simulink library "MESSIN_Library"  (R2024a)
settings: Solver=VariableStepAuto  StartTime=0.0  StopTime=10.0  RelTol=1e-3
undefined symbols (not defined in the file or in its folder): actuatorCommand, commandedActuator, commandMode, externCommand, ready, remoteControlDevice, sensor, supervisor, timestampUTC, useXNAllocation
libraries: $bdroot x376, etargetslib x52, simulink x19
(part 2 of 5)

== system MESSIN_Library/State Message/Empty MESSIN State Bus/Empty INS Bus ==
  Bus Creator1 : BusCreator  Inputs=5
  Bus Creator2 : BusCreator  Inputs=17
  Constant1 : Constant  Value=0  OutDataTypeStr=uint8
  Constant{2..8,12..14,18..23} (16 alike) : Constant  Value=0.0  OutDataTypeStr=double
  Constant24 : Constant  Value=false  OutDataTypeStr=boolean
  Constant25 : Constant  Value=false  OutDataTypeStr=boolean
  Constant26 : Constant  Value=0  OutDataTypeStr=uint16
  Constant27 : Constant  Value=0  OutDataTypeStr=uint16
  Signal Specification1 : SignalSpecification  OutDataTypeStr=double  Unit=s  Dimensions=1
  Signal Specification{2..3,11..13} (5 alike) : SignalSpecification  OutDataTypeStr=double  Unit=rad  Dimensions=1
  Signal Specification17 : SignalSpecification  OutDataTypeStr=double  Unit=rad/s  Dimensions=1
  Signal Specification18 : SignalSpecification  OutDataTypeStr=double  Unit=rad/s  Dimensions=1
  Signal Specification19 : SignalSpecification  OutDataTypeStr=double  Unit=rad/s  Dimensions=1
  Signal Specification20 : SignalSpecification  OutDataTypeStr=double  Unit=m/s^2  Dimensions=1
  Signal Specification21 : SignalSpecification  OutDataTypeStr=double  Unit=m/s^2  Dimensions=1
  Signal Specification22 : SignalSpecification  OutDataTypeStr=double  Unit=m/s^2  Dimensions=1
  Signal Specification23 : SignalSpecification  OutDataTypeStr=uint8  Dimensions=1
  Signal Specification24 : SignalSpecification  OutDataTypeStr=boolean  Dimensions=1
  Signal Specification25 : SignalSpecification  OutDataTypeStr=boolean  Dimensions=1
  Signal Specification26 : SignalSpecification  OutDataTypeStr=uint16  Dimensions=1
  Signal Specification27 : SignalSpecification  OutDataTypeStr=uint16  Dimensions=1
  Signal Specification4 : SignalSpecification  OutDataTypeStr=double  Unit=m  Dimensions=1
  Signal Specification5 : SignalSpecification  OutDataTypeStr=double  Unit=m/s  Dimensions=1
  Signal Specification6 : SignalSpecification  OutDataTypeStr=double  Unit=m/s  Dimensions=1
  Signal Specification7 : SignalSpecification  OutDataTypeStr=double  Unit=m/s  Dimensions=1
  insLFK100 : Outport
  wires:
  Signal Specification1/1 -> Bus Creator2/1  "timestampUTC"
  Signal Specification6/1 -> Bus Creator2/6  "velocityEast"
  Constant4/1 -> Signal Specification3/1
  Constant19/1 -> Signal Specification18/1
  Signal Specification20/1 -> Bus Creator2/14  "bodyAccelerationX"
  Constant23/1 -> Signal Specification22/1
  Signal Specification13/1 -> Bus Creator2/10  "heading"
  Signal Specification2/1 -> Bus Creator2/2  "latitude"
  Constant14/1 -> Signal Specification13/1
  Bus Creator2/1 -> insLFK100/1
  Constant6/1 -> Signal Specification5/1
  Constant13/1 -> Signal Specification12/1
  Signal Specification11/1 -> Bus Creator2/8  "roll"
  Constant3/1 -> Signal Specification2/1
  Signal Specification12/1 -> Bus Creator2/9  "pitch"
  Signal Specification5/1 -> Bus Creator2/5  "velocityNorth"
  Signal Specification18/1 -> Bus Creator2/12  "bodyAngularRateY"
  Constant5/1 -> Signal Specification4/1
  Constant18/1 -> Signal Specification17/1
  Signal Specification3/1 -> Bus Creator2/3  "longitude"
  Signal Specification4/1 -> Bus Creator2/4  "heave"
  Constant20/1 -> Signal Specification19/1
  Constant12/1 -> Signal Specification11/1
  Constant2/1 -> Signal Specification1/1
  Signal Specification22/1 -> Bus Creator2/16  "bodyAccelerationZ"
  Signal Specification7/1 -> Bus Creator2/7  "velocityDown"
  Signal Specification19/1 -> Bus Creator2/13  "bodyAngularRateZ"
  Constant8/1 -> Signal Specification7/1
  Constant21/1 -> Signal Specification20/1
  Constant22/1 -> Signal Specification21/1
  Constant7/1 -> Signal Specification6/1
  Signal Specification17/1 -> Bus Creator2/11  "bodyAngularRateX"
  Signal Specification21/1 -> Bus Creator2/15  "bodyAccelerationY"
  Constant1/1 -> Signal Specification23/1
  Signal Specification27/1 -> Bus Creator1/5  "statusWord2"
  Signal Specification26/1 -> Bus Creator1/4  "statusWord1"
  Signal Specification25/1 -> Bus Creator1/3  "reducedAccuracy"
  Signal Specification24/1 -> Bus Creator1/2  "systemFailure"
  Signal Specification23/1 -> Bus Creator1/1  "mode"
  Constant24/1 -> Signal Specification24/1
  Constant25/1 -> Signal Specification25/1
  Constant26/1 -> Signal Specification26/1
  Constant27/1 -> Signal Specification27/1
  Bus Creator1/1 -> Bus Creator2/17  "details"

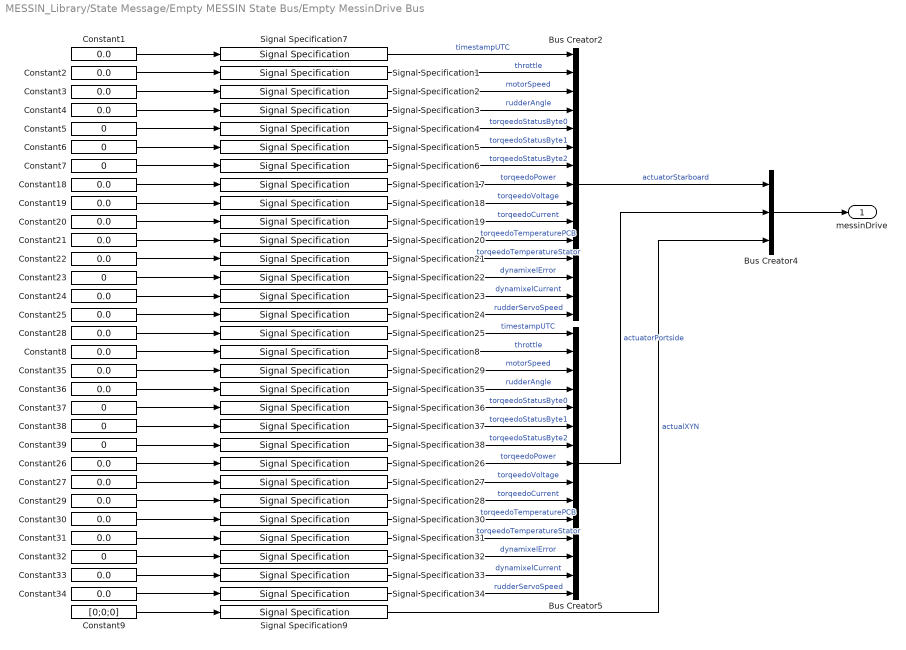
== system MESSIN_Library/State Message/Empty MESSIN State Bus/Empty MessinDrive Bus ==
  Bus Creator2 : BusCreator  Inputs=15
  Bus Creator4 : BusCreator  Inputs=3
  Bus Creator5 : BusCreator  Inputs=15
  Constant{1..4,8,18..22,24..31,33..36} (22 alike) : Constant  Value=0.0  OutDataTypeStr=double
  Constant{5..7,23,32,37..39} (8 alike) : Constant  Value=0  OutDataTypeStr=uint8
  Constant9 : Constant  Value=[0;0;0]  OutDataTypeStr=double
  Signal Specification1 : SignalSpecification  OutDataTypeStr=double  Unit=1  Dimensions=1
  Signal Specification17 : SignalSpecification  OutDataTypeStr=double  Unit=W  Dimensions=1
  Signal Specification18 : SignalSpecification  OutDataTypeStr=double  Unit=V  Dimensions=1
  Signal Specification{19,23,28,33} (4 alike) : SignalSpecification  OutDataTypeStr=double  Unit=A  Dimensions=1
  Signal Specification{2,24,29,34} (4 alike) : SignalSpecification  OutDataTypeStr=double  Unit=rad/s  Dimensions=1
  Signal Specification{20..21,30..31} (4 alike) : SignalSpecification  OutDataTypeStr=double  Unit=°C  Dimensions=1
  Signal Specification{4..6,22,32,36..38} (8 alike) : SignalSpecification  OutDataTypeStr=uint8  Unit=1  Dimensions=1
  Signal Specification25 : SignalSpecification  OutDataTypeStr=double  Unit=s  Dimensions=1
  Signal Specification26 : SignalSpecification  OutDataTypeStr=double  Unit=W  Dimensions=1
  Signal Specification27 : SignalSpecification  OutDataTypeStr=double  Unit=V  Dimensions=1
  Signal Specification3 : SignalSpecification  OutDataTypeStr=double  Unit=rad  Dimensions=1
  Signal Specification35 : SignalSpecification  OutDataTypeStr=double  Unit=rad  Dimensions=1
  Signal Specification7 : SignalSpecification  OutDataTypeStr=double  Unit=s  Dimensions=1
  Signal Specification8 : SignalSpecification  OutDataTypeStr=double  Unit=1  Dimensions=1
  Signal Specification9 : SignalSpecification  OutDataTypeStr=double  Dimensions=3
  messinDrive : Outport
  wires:
  Constant36/1 -> Signal Specification35/1
  Signal Specification1/1 -> Bus Creator2/2  "throttle"
  Signal Specification17/1 -> Bus Creator2/8  "torqeedoPower"
  Constant20/1 -> Signal Specification19/1
  Constant30/1 -> Signal Specification30/1
  Constant37/1 -> Signal Specification36/1
  Signal Specification25/1 -> Bus Creator5/1  "timestampUTC"
  Signal Specification4/1 -> Bus Creator2/5  "torqeedoStatusByte0"
  Signal Specification26/1 -> Bus Creator5/8  "torqeedoPower"
  Signal Specification2/1 -> Bus Creator2/3  "motorSpeed"
  Constant22/1 -> Signal Specification21/1
  Constant18/1 -> Signal Specification17/1
  Signal Specification5/1 -> Bus Creator2/6  "torqeedoStatusByte1"
  Constant25/1 -> Signal Specification24/1
  Signal Specification37/1 -> Bus Creator5/6  "torqeedoStatusByte1"
  Signal Specification21/1 -> Bus Creator2/12  "torqeedoTemperatureStator"
  Constant32/1 -> Signal Specification32/1
  Signal Specification36/1 -> Bus Creator5/5  "torqeedoStatusByte0"
  Constant2/1 -> Signal Specification1/1
  Constant5/1 -> Signal Specification4/1
  Signal Specification28/1 -> Bus Creator5/10  "torqeedoCurrent"
  Constant35/1 -> Signal Specification29/1
  Signal Specification19/1 -> Bus Creator2/10  "torqeedoCurrent"
  Signal Specification32/1 -> Bus Creator5/13  "dynamixelError"
  Constant7/1 -> Signal Specification6/1
  Constant21/1 -> Signal Specification20/1
  Signal Specification29/1 -> Bus Creator5/3  "motorSpeed"
  Signal Specification30/1 -> Bus Creator5/11  "torqeedoTemperaturePCB"
  Signal Specification38/1 -> Bus Creator5/7  "torqeedoStatusByte2"
  Bus Creator4/1 -> messinDrive/1
  Signal Specification22/1 -> Bus Creator2/13  "dynamixelError"
  Constant4/1 -> Signal Specification3/1
  Signal Specification35/1 -> Bus Creator5/4  "rudderAngle"
  Constant28/1 -> Signal Specification25/1
  Signal Specification20/1 -> Bus Creator2/11  "torqeedoTemperaturePCB"
  Signal Specification24/1 -> Bus Creator2/15  "rudderServoSpeed"
  Constant24/1 -> Signal Specification23/1
  Constant19/1 -> Signal Specification18/1
  Constant27/1 -> Signal Specification27/1
  Constant6/1 -> Signal Specification5/1
  Constant33/1 -> Signal Specification33/1
  Signal Specification18/1 -> Bus Creator2/9  "torqeedoVoltage"
  Constant29/1 -> Signal Specification28/1
  Signal Specification3/1 -> Bus Creator2/4  "rudderAngle"
  Bus Creator2/1 -> Bus Creator4/1  "actuatorStarboard"
  Constant3/1 -> Signal Specification2/1
  Constant31/1 -> Signal Specification31/1
  Signal Specification6/1 -> Bus Creator2/7  "torqeedoStatusByte2"
  Constant39/1 -> Signal Specification38/1
  Constant26/1 -> Signal Specification26/1
  Constant38/1 -> Signal Specification37/1
  Signal Specification34/1 -> Bus Creator5/15  "rudderServoSpeed"
  Constant23/1 -> Signal Specification22/1
  Signal Specification23/1 -> Bus Creator2/14  "dynamixelCurrent"
  Bus Creator5/1 -> Bus Creator4/2  "actuatorPortside"
  Signal Specification31/1 -> Bus Creator5/12  "torqeedoTemperatureStator"
  Signal Specification33/1 -> Bus Creator5/14  "dynamixelCurrent"
  Constant34/1 -> Signal Specification34/1
  Signal Specification27/1 -> Bus Creator5/9  "torqeedoVoltage"
  Constant1/1 -> Signal Specification7/1
  Signal Specification7/1 -> Bus Creator2/1  "timestampUTC"
  Constant8/1 -> Signal Specification8/1
  Signal Specification8/1 -> Bus Creator5/2  "throttle"
  Constant9/1 -> Signal Specification9/1
  Signal Specification9/1 -> Bus Creator4/3  "actualXYN"

== system MESSIN_Library/State Message/Empty MESSIN State Bus/Empty Navigation Bus ==
  Bus Creator5 : BusCreator  Inputs=16
  Bus Creator6 : BusCreator  Inputs=3
  Bus Creator7 : BusCreator  Inputs=1
  Constant{,1..4,9..13,17..18,20,23..26} (17 alike) : Constant  Value=0.0  OutDataTypeStr=double
  Constant19 : Constant  Value=false  OutDataTypeStr=boolean
  Signal Specification{1,3,8..9,24..26} (7 alike) : SignalSpecification  OutDataTypeStr=double  Unit=rad  Dimensions=1
  Signal Specification{2,4,10..12} (5 alike) : SignalSpecification  OutDataTypeStr=double  Unit=m/s  Dimensions=1
  Signal Specification13 : SignalSpecification  OutDataTypeStr=double  Unit=rad/s  Dimensions=1
  Signal Specification17 : SignalSpecification  OutDataTypeStr=double  Unit=s  Dimensions=1
  Signal Specification18 : SignalSpecification  OutDataTypeStr=boolean  Unit=1  Dimensions=1
  Signal Specification19 : SignalSpecification  OutDataTypeStr=double  Unit=rad/s  Dimensions=1
  Signal Specification20 : SignalSpecification  OutDataTypeStr=double  Unit=rad/s  Dimensions=1
  Signal Specification23 : SignalSpecification  OutDataTypeStr=double  Unit=m  Dimensions=1
  navigation : Outport
  wires:
  Signal Specification25/1 -> Bus Creator5/5  "orientationPitch"
  Signal Specification23/1 -> Bus Creator5/3  "positionAltitude"
  Signal Specification20/1 -> Bus Creator5/12  "velocityR"
  Constant25/1 -> Signal Specification25/1
  Constant20/1 -> Signal Specification11/1
  Constant18/1 -> Signal Specification10/1
  Signal Specification19/1 -> Bus Creator5/11  "velocityQ"
  Constant24/1 -> Signal Specification24/1
  Bus Creator7/1 -> Bus Creator6/2  "info"
  Signal Specification10/1 -> Bus Creator5/7  "velocityU"
  Constant11/1 -> Signal Specification13/1
  Constant10/1 -> Signal Specification12/1
  Constant23/1 -> Signal Specification23/1
  Bus Creator6/1 -> navigation/1
  Signal Specification24/1 -> Bus Creator5/4  "orientationRoll"
  Signal Specification13/1 -> Bus Creator5/10  "velocityP"
  Signal Specification26/1 -> Bus Creator5/6  "orientationYaw"
  Signal Specification8/1 -> Bus Creator5/1  "positionLatitude"
  Constant26/1 -> Signal Specification26/1
  Constant19/1 -> Signal Specification18/1
  Signal Specification12/1 -> Bus Creator5/9  "velocityW"
  Constant13/1 -> Signal Specification20/1
  Constant9/1 -> Signal Specification9/1
  Constant12/1 -> Signal Specification19/1
  Signal Specification9/1 -> Bus Creator5/2  "positionLongitude"
  Signal Specification18/1 -> Bus Creator7/1  "valid"
  Signal Specification17/1 -> Bus Creator6/1  "timestampUTC"
  Bus Creator5/1 -> Bus Creator6/3  "state"
  Constant/1 -> Signal Specification8/1
  Constant17/1 -> Signal Specification17/1
  Signal Specification11/1 -> Bus Creator5/8  "velocityV"
  Constant1/1 -> Signal Specification1/1
  Signal Specification1/1 -> Bus Creator5/13  "courseOverGround"
  Constant2/1 -> Signal Specification2/1
  Signal Specification2/1 -> Bus Creator5/14  "speedOverGround"
  Constant4/1 -> Signal Specification4/1
  Constant3/1 -> Signal Specification3/1
  Signal Specification3/1 -> Bus Creator5/15  "absoluteWindAngle"
  Signal Specification4/1 -> Bus Creator5/16  "absoluteWindSpeed"

== system MESSIN_Library/State Message/Empty MESSIN State Bus/Empty RCD Bus ==
  Bus Creator2 : BusCreator  Inputs=3
  Constant1 : Constant  Value=[0.0; 0.0; 0.0]  OutDataTypeStr=double
  Constant2 : Constant  Value=0.0  OutDataTypeStr=double
  Constant3 : Constant  Value=[0.0; 0.0; 0.0]  OutDataTypeStr=double
  Signal Specification1 : SignalSpecification  OutDataTypeStr=double  Unit=s  Dimensions=1
  Signal Specification2 : SignalSpecification  OutDataTypeStr=double  Unit=1  Dimensions=3
  Signal Specification3 : SignalSpecification  OutDataTypeStr=double  Unit=1  Dimensions=3
  rcd : Outport
  wires:
  Bus Creator2/1 -> rcd/1
  Constant3/1 -> Signal Specification2/1
  Signal Specification3/1 -> Bus Creator2/3  "joystickRight"
  Constant1/1 -> Signal Specification3/1
  Constant2/1 -> Signal Specification1/1
  Signal Specification2/1 -> Bus Creator2/2  "joystickLeft"
  Signal Specification1/1 -> Bus Creator2/1  "timestampUTC"

== system MESSIN_Library/State Message/Empty MESSIN State Bus/Empty Supervisor Bus ==
  Bus Creator2 : BusCreator  Inputs=6
  Constant{2..6} (5 alike) : Constant  Value=false  OutDataTypeStr=boolean
  Constant7 : Constant  Value=0  OutDataTypeStr=uint8
  Signal Specification{1..5} (5 alike) : SignalSpecification  OutDataTypeStr=boolean  Unit=1  Dimensions=1
  Signal Specification6 : SignalSpecification  OutDataTypeStr=uint8  Unit=1  Dimensions=1
  supervisor : Outport
  wires:
  Bus Creator2/1 -> supervisor/1
  Constant5/1 -> Signal Specification4/1
  Constant4/1 -> Signal Specification3/1
  Constant2/1 -> Signal Specification2/1
  Signal Specification5/1 -> Bus Creator2/5  "externModeEnabled"
  Signal Specification1/1 -> Bus Creator2/1  "torqeedoPoweredOn"
  Signal Specification4/1 -> Bus Creator2/4  "actuatorsSynchronized"
  Constant6/1 -> Signal Specification5/1
  Signal Specification6/1 -> Bus Creator2/6  "internalOperationMode"
  Constant3/1 -> Signal Specification1/1
  Constant7/1 -> Signal Specification6/1
  Signal Specification2/1 -> Bus Creator2/2  "actuatorsEnabled"
  Signal Specification3/1 -> Bus Creator2/3  "lightEnabled"

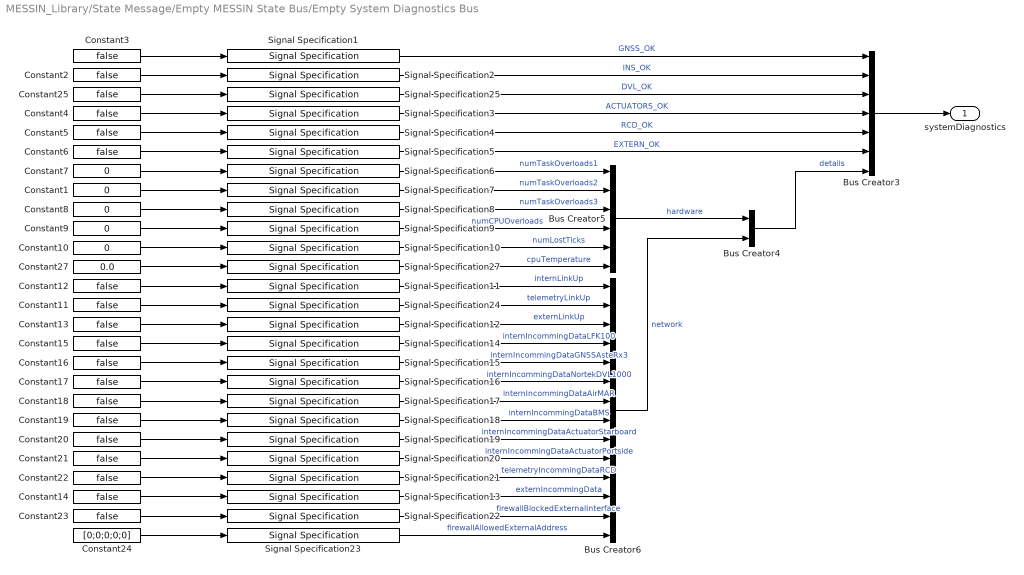
== system MESSIN_Library/State Message/Empty MESSIN State Bus/Empty System Diagnostics Bus ==
  Bus Creator3 : BusCreator  Inputs=7
  Bus Creator4 : BusCreator  Inputs=2
  Bus Creator5 : BusCreator  Inputs=6
  Bus Creator6 : BusCreator  Inputs=14
  Constant{1,7..10} (5 alike) : Constant  Value=0  OutDataTypeStr=uint32
  Constant{2..6,11..23,25} (19 alike) : Constant  Value=false  OutDataTypeStr=boolean
  Constant24 : Constant  Value=[0;0;0;0;0]  OutDataTypeStr=uint16
  Constant27 : Constant  Value=0.0  OutDataTypeStr=double
  Signal Specification{1..5,11..22,24..25} (19 alike) : SignalSpecification  OutDataTypeStr=boolean  Unit=1  Dimensions=1
  Signal Specification{6..10} (5 alike) : SignalSpecification  OutDataTypeStr=uint32  Unit=1  Dimensions=1
  Signal Specification23 : SignalSpecification  OutDataTypeStr=uint16  Unit=1  Dimensions=5
  Signal Specification27 : SignalSpecification  OutDataTypeStr=double  Unit=°C  Dimensions=1
  systemDiagnostics : Outport
  wires:
  Signal Specification11/1 -> Bus Creator6/1  "internLinkUp"
  Signal Specification12/1 -> Bus Creator6/3  "externLinkUp"
  Signal Specification10/1 -> Bus Creator5/5  "numLostTicks"
  Constant5/1 -> Signal Specification4/1
  Signal Specification18/1 -> Bus Creator6/8  "internIncommingDataBMS"
  Signal Specification21/1 -> Bus Creator6/11  "telemetryIncommingDataRCD"
  Signal Specification22/1 -> Bus Creator6/13  "firewallBlockedExternalInterface"
  Signal Specification16/1 -> Bus Creator6/6  "internIncommingDataNortekDVL1000"
  Constant6/1 -> Signal Specification5/1
  Signal Specification19/1 -> Bus Creator6/9  "internIncommingDataActuatorStarboard"
  Signal Specification6/1 -> Bus Creator5/1  "numTaskOverloads1"
  Bus Creator3/1 -> systemDiagnostics/1
  Constant3/1 -> Signal Specification1/1
  Constant7/1 -> Signal Specification6/1
  Constant18/1 -> Signal Specification17/1
  Constant19/1 -> Signal Specification18/1
  Signal Specification3/1 -> Bus Creator3/4  "ACTUATORS_OK"
  Bus Creator4/1 -> Bus Creator3/7  "details"
  Bus Creator6/1 -> Bus Creator4/2  "network"
  Signal Specification20/1 -> Bus Creator6/10  "internIncommingDataActuatorPortside"
  Signal Specification23/1 -> Bus Creator6/14  "firewallAllowedExternalAddress"
  Constant13/1 -> Signal Specification12/1
  Constant21/1 -> Signal Specification20/1
  Constant4/1 -> Signal Specification3/1
  Constant24/1 -> Signal Specification23/1
  Signal Specification5/1 -> Bus Creator3/6  "EXTERN_OK"
  Constant22/1 -> Signal Specification21/1
  Signal Specification8/1 -> Bus Creator5/3  "numTaskOverloads3"
  Signal Specification2/1 -> Bus Creator3/2  "INS_OK"
  Constant15/1 -> Signal Specification14/1
  Signal Specification14/1 -> Bus Creator6/4  "internIncommingDataLFK100"
  Signal Specification9/1 -> Bus Creator5/4  "numCPUOverloads"
  Bus Creator5/1 -> Bus Creator4/1  "hardware"
  Constant17/1 -> Signal Specification16/1
  Constant23/1 -> Signal Specification22/1
  Constant20/1 -> Signal Specification19/1
  Constant12/1 -> Signal Specification11/1
  Constant14/1 -> Signal Specification13/1
  Signal Specification4/1 -> Bus Creator3/5  "RCD_OK"
  Signal Specification7/1 -> Bus Creator5/2  "numTaskOverloads2"
  Signal Specification17/1 -> Bus Creator6/7  "internIncommingDataAirMAR"
  Constant16/1 -> Signal Specification15/1
  Signal Specification15/1 -> Bus Creator6/5  "internIncommingDataGNSSAsteRx3"
  Constant2/1 -> Signal Specification2/1
  Signal Specification1/1 -> Bus Creator3/1  "GNSS_OK"
  Constant1/1 -> Signal Specification7/1
  Constant8/1 -> Signal Specification8/1
  Constant9/1 -> Signal Specification9/1
  Constant10/1 -> Signal Specification10/1
  Signal Specification13/1 -> Bus Creator6/12  "externIncommingData"
  Constant11/1 -> Signal Specification24/1
  Signal Specification24/1 -> Bus Creator6/2  "telemetryLinkUp"
  Constant25/1 -> Signal Specification25/1
  Signal Specification25/1 -> Bus Creator3/3  "DVL_OK"
  Constant27/1 -> Signal Specification27/1
  Signal Specification27/1 -> Bus Creator5/6  "cpuTemperature"

== system MESSIN_Library/State Message/Pack MESSIN State Message/Pack AirMAR ==
  airMAR : Inport
  Bus Selector1 : BusSelector  OutputSignals=air
  Bus Selector2 : BusSelector  OutputSignals=timestampUTC,pressure,airTemperature
  Bus Selector3 : BusSelector  OutputSignals=relativeWind
  Bus Selector4 : BusSelector  OutputSignals=timestampUTC,windAngle,windSpeed
  Byte Pack1 : S-Function  FunctionName=any2byte  Parameters=datatypesout,byteAlign  SFunctionDeploymentMode=off  EnableBusSupport=off  mask(Byte pack){datatypes={'double','single','single'}, byteAlign=1}
      mask prompts: datatypes "Input port data types (cell array):"; byteAlign "Byte alignment:"
      mask help: Pack input data into a single output vector of type uint8. Insert before a UDP Send block to produce a uint8 byte vector from multiple vectors of varying data type.
      mask init:
      | datatypesout = bytepack_callback(datatypes);
      settings: LibrarySourceBlock=embeddedtargetslib/Host Communication/Byte Pack
      mask Help: eval('linkfoundation.util.openBlockHelp(''etargetslibbytepack'')');
      mask TypeOptions byteAlign: 1 | 2 | 4 | 8
      mask Display:
      | color('blue');
      | text(0.95, 0.90, '', ...
      |                 'horizontalalignment', 'right');
      | color('black');
      | text(0.50, 0.12, 'Byte Pack', ...
      |                 'horizontalAlignment','center');
  Byte Pack2 : $bdroot/State Message/Pack MESSIN State Message/Pack AirMAR/Byte Pack1  datatypes={'double','single','single'}  byteAlign=1
      settings: LibrarySourceBlock=embeddedtargetslib/Host Communication/Byte Pack
  Convert Double Network Byte Order : $bdroot/Utilities/Convert Double Network Byte Order
  Convert Double Network Byte Order1 : $bdroot/Utilities/Convert Double Network Byte Order
  Convert Single Network Byte Order{,1..3} (4 alike) : $bdroot/Utilities/Convert Single Network Byte Order
  Data Type Conversion1 : DataTypeConversion  OutDataTypeStr=double  SaturateOnIntegerOverflow=off  RndMeth=Floor
  Data Type Conversion{2..3,5..6} (4 alike) : DataTypeConversion  OutDataTypeStr=single  SaturateOnIntegerOverflow=off  RndMeth=Floor
  Data Type Conversion4 : DataTypeConversion  OutDataTypeStr=double  SaturateOnIntegerOverflow=off  RndMeth=Floor
  Vector Concatenate : Concatenate
  bytes : Outport
  wires:
  Vector Concatenate/1 -> bytes/1
  airMAR/1 -> Bus Selector3/1, Bus Selector1/1
  Bus Selector2/3 -> Data Type Conversion3/1  "<airTemperature>"
  Bus Selector2/2 -> Data Type Conversion2/1  "<pressure>"
  Bus Selector2/1 -> Data Type Conversion1/1  "<timestampUTC>"
  Convert Double Network Byte Order/1 -> Byte Pack1/1
  Data Type Conversion1/1 -> Convert Double Network Byte Order/1
  Bus Selector1/1 -> Bus Selector2/1  "<air>"
  Byte Pack1/1 -> Vector Concatenate/1
  Bus Selector3/1 -> Bus Selector4/1  "<relativeWind>"
  Bus Selector4/1 -> Data Type Conversion4/1  "<timestampUTC>"
  Bus Selector4/2 -> Data Type Conversion5/1  "<windAngle>"
  Bus Selector4/3 -> Data Type Conversion6/1  "<windSpeed>"
  Byte Pack2/1 -> Vector Concatenate/2
  Convert Single Network Byte Order/1 -> Byte Pack1/2
  Data Type Conversion2/1 -> Convert Single Network Byte Order/1
  Data Type Conversion3/1 -> Convert Single Network Byte Order1/1
  Convert Single Network Byte Order1/1 -> Byte Pack1/3
  Convert Single Network Byte Order3/1 -> Byte Pack2/3
  Data Type Conversion6/1 -> Convert Single Network Byte Order3/1
  Data Type Conversion5/1 -> Convert Single Network Byte Order2/1
  Convert Single Network Byte Order2/1 -> Byte Pack2/2
  Data Type Conversion4/1 -> Convert Double Network Byte Order1/1
  Convert Double Network Byte Order1/1 -> Byte Pack2/1

== system MESSIN_Library/State Message/Pack MESSIN State Message/Pack BMS ==
  bms : Inport
  Bus Selector : BusSelector  OutputSignals=batteryStarboard
  Bus Selector1 : BusSelector  OutputSignals=timestampUTC,voltage,current,consumedElectricCharge,stateOfCharge
  Bus Selector19 : BusSelector  OutputSignals=timestampUTC,voltage,current,consumedElectricCharge,stateOfCharge
  Bus Selector2 : BusSelector  OutputSignals=batteryPortside
  Byte Pack : etargetslib/Byte Pack  datatypes={'double','single','single','single','single'}  byteAlign=1
  Byte Pack1 : etargetslib/Byte Pack  datatypes={'double','single','single','single','single'}  byteAlign=1
  Convert Double Network Byte Order1 : $bdroot/Utilities/Convert Double Network Byte Order
  Convert Double Network Byte Order2 : $bdroot/Utilities/Convert Double Network Byte Order
  Convert Single Network Byte Order{1..8} (8 alike) : $bdroot/Utilities/Convert Single Network Byte Order
  Data Type Conversion : DataTypeConversion  OutDataTypeStr=double  SaturateOnIntegerOverflow=off  RndMeth=Floor
  Data Type Conversion{1,3..6,9..10,50} (8 alike) : DataTypeConversion  OutDataTypeStr=single  SaturateOnIntegerOverflow=off  RndMeth=Floor
  Data Type Conversion2 : DataTypeConversion  OutDataTypeStr=double  SaturateOnIntegerOverflow=off  RndMeth=Floor
  Vector Concatenate : Concatenate
  bytes : Outport
  wires:
  Data Type Conversion10/1 -> Convert Single Network Byte Order3/1
  Data Type Conversion9/1 -> Convert Single Network Byte Order2/1
  Convert Single Network Byte Order3/1 -> Byte Pack/4
  Convert Single Network Byte Order2/1 -> Byte Pack/3
  Bus Selector19/4 -> Data Type Conversion10/1  "<consumedElectricCharge>"
  Bus Selector19/3 -> Data Type Conversion9/1  "<current>"
  Data Type Conversion50/1 -> Convert Single Network Byte Order1/1
  Bus Selector19/2 -> Data Type Conversion50/1  "<voltage>"
  Bus Selector19/1 -> Data Type Conversion/1  "<timestampUTC>"
  Bus Selector/1 -> Bus Selector19/1  "<batteryStarboard>"
  bms/1 -> Bus Selector2/1, Bus Selector/1
  Vector Concatenate/1 -> bytes/1
  Byte Pack/1 -> Vector Concatenate/1
  Convert Double Network Byte Order1/1 -> Byte Pack/1
  Data Type Conversion/1 -> Convert Double Network Byte Order1/1
  Convert Single Network Byte Order1/1 -> Byte Pack/2
  Bus Selector19/5 -> Data Type Conversion1/1  "<stateOfCharge>"
  Data Type Conversion1/1 -> Convert Single Network Byte Order4/1
  Convert Single Network Byte Order4/1 -> Byte Pack/5
  Convert Single Network Byte Order8/1 -> Byte Pack1/5
  Data Type Conversion3/1 -> Convert Single Network Byte Order8/1
  Bus Selector1/5 -> Data Type Conversion3/1  "<stateOfCharge>"
  Convert Single Network Byte Order5/1 -> Byte Pack1/2
  Data Type Conversion2/1 -> Convert Double Network Byte Order2/1
  Convert Double Network Byte Order2/1 -> Byte Pack1/1
  Bus Selector2/1 -> Bus Selector1/1  "<batteryPortside>"
  Bus Selector1/1 -> Data Type Conversion2/1  "<timestampUTC>"
  Bus Selector1/2 -> Data Type Conversion5/1  "<voltage>"
  Data Type Conversion5/1 -> Convert Single Network Byte Order5/1
  Bus Selector1/3 -> Data Type Conversion6/1  "<current>"
  Bus Selector1/4 -> Data Type Conversion4/1  "<consumedElectricCharge>"
  Convert Single Network Byte Order6/1 -> Byte Pack1/3
  Convert Single Network Byte Order7/1 -> Byte Pack1/4
  Data Type Conversion6/1 -> Convert Single Network Byte Order6/1
  Data Type Conversion4/1 -> Convert Single Network Byte Order7/1
  Byte Pack1/1 -> Vector Concatenate/2

== system MESSIN_Library/State Message/Pack MESSIN State Message/Pack CommandedActuator ==
  commandedActuator : Inport
  Bus Selector2 : BusSelector  OutputSignals=throttleStarboard,throttlePortside,angleStarboard,anglePortside
  Byte Pack : etargetslib/Byte Pack  datatypes={'double','double','double','double'}  byteAlign=1
  Convert Double Network Byte Order{1..4} (4 alike) : $bdroot/Utilities/Convert Double Network Byte Order
  Data Type Conversion{,1..3} (4 alike) : DataTypeConversion  OutDataTypeStr=double  SaturateOnIntegerOverflow=off  RndMeth=Floor
  bytes : Outport
  wires:
  Convert Double Network Byte Order4/1 -> Byte Pack/4
  Convert Double Network Byte Order3/1 -> Byte Pack/3
  Convert Double Network Byte Order2/1 -> Byte Pack/2
  Convert Double Network Byte Order1/1 -> Byte Pack/1
  Bus Selector2/4 -> Data Type Conversion3/1  "<anglePortside>"
  Bus Selector2/3 -> Data Type Conversion2/1  "<angleStarboard>"
  Data Type Conversion3/1 -> Convert Double Network Byte Order4/1
  Data Type Conversion2/1 -> Convert Double Network Byte Order3/1
  Bus Selector2/2 -> Data Type Conversion1/1  "<throttlePortside>"
  Data Type Conversion1/1 -> Convert Double Network Byte Order2/1
  Bus Selector2/1 -> Data Type Conversion/1  "<throttleStarboard>"
  commandedActuator/1 -> Bus Selector2/1
  Data Type Conversion/1 -> Convert Double Network Byte Order1/1
  Byte Pack/1 -> bytes/1

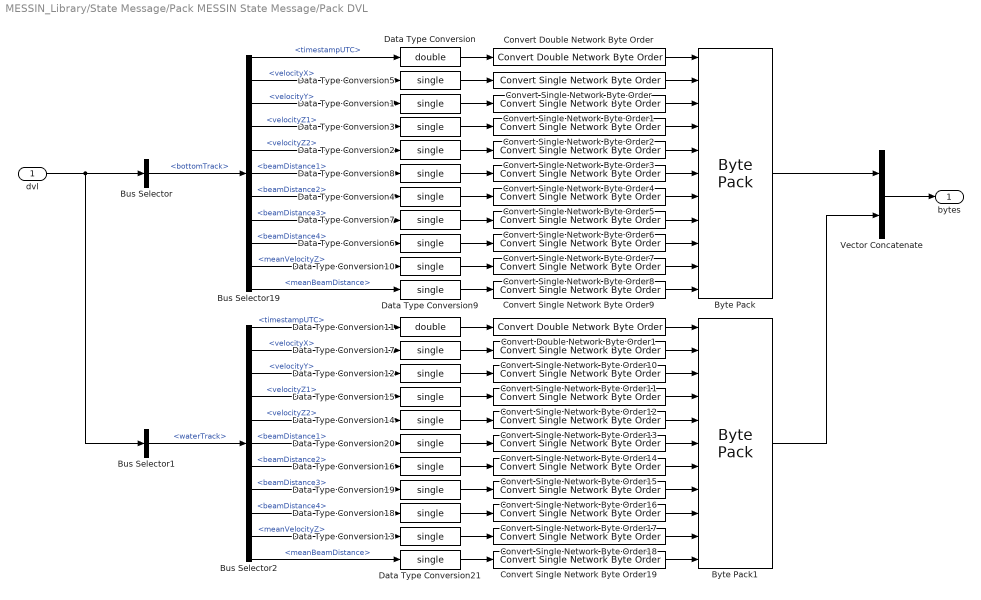
== system MESSIN_Library/State Message/Pack MESSIN State Message/Pack DVL ==
  dvl : Inport
  Bus Selector : BusSelector  OutputSignals=bottomTrack
  Bus Selector1 : BusSelector  OutputSignals=waterTrack
  Bus Selector19 : BusSelector  OutputSignals=timestampUTC,velocityX,velocityY,velocityZ1,velocityZ2,beamDistance1,beamDistance2,beamDistance3,beamDistance4,meanVelocityZ,meanBeamDistance
  Bus Selector2 : BusSelector  OutputSignals=timestampUTC,velocityX,velocityY,velocityZ1,velocityZ2,beamDistance1,beamDistance2,beamDistance3,beamDistance4,meanVelocityZ,meanBeamDistance
  Byte Pack : etargetslib/Byte Pack  datatypes={'double','single','single','single','single','single','single','single','single','single','single'}  byteAlign=1
  Byte Pack1 : etargetslib/Byte Pack  datatypes={'double','single','single','single','single','single','single','single','single','single','single'}  byteAlign=1
  Convert Double Network Byte Order : $bdroot/Utilities/Convert Double Network Byte Order
  Convert Double Network Byte Order1 : $bdroot/Utilities/Convert Double Network Byte Order
  Convert Single Network Byte Order{,1..19} (20 alike) : $bdroot/Utilities/Convert Single Network Byte Order
  Data Type Conversion : DataTypeConversion  OutDataTypeStr=double  SaturateOnIntegerOverflow=off  RndMeth=Floor
  Data Type Conversion{1..10,12..21} (20 alike) : DataTypeConversion  OutDataTypeStr=single  SaturateOnIntegerOverflow=off  RndMeth=Floor
  Data Type Conversion11 : DataTypeConversion  OutDataTypeStr=double  SaturateOnIntegerOverflow=off  RndMeth=Floor
  Vector Concatenate : Concatenate
  bytes : Outport
  wires:
  Data Type Conversion/1 -> Convert Double Network Byte Order/1
  Convert Double Network Byte Order/1 -> Byte Pack/1
  Byte Pack/1 -> Vector Concatenate/1
  Vector Concatenate/1 -> bytes/1
  dvl/1 -> Bus Selector1/1, Bus Selector/1
  Bus Selector/1 -> Bus Selector19/1  "<bottomTrack>"
  Bus Selector19/1 -> Data Type Conversion/1  "<timestampUTC>"
  Bus Selector19/2 -> Data Type Conversion5/1  "<velocityX>"
  Bus Selector19/3 -> Data Type Conversion1/1  "<velocityY>"
  Bus Selector19/4 -> Data Type Conversion3/1  "<velocityZ1>"
  Bus Selector1/1 -> Bus Selector2/1  "<waterTrack>"
  Bus Selector19/8 -> Data Type Conversion7/1  "<beamDistance3>"
  Bus Selector19/7 -> Data Type Conversion4/1  "<beamDistance2>"
  Bus Selector19/6 -> Data Type Conversion8/1  "<beamDistance1>"
  Bus Selector19/5 -> Data Type Conversion2/1  "<velocityZ2>"
  Bus Selector19/9 -> Data Type Conversion6/1  "<beamDistance4>"
  Bus Selector19/10 -> Data Type Conversion10/1  "<meanVelocityZ>"
  Bus Selector19/11 -> Data Type Conversion9/1  "<meanBeamDistance>"
  Bus Selector2/11 -> Data Type Conversion21/1  "<meanBeamDistance>"
  Bus Selector2/10 -> Data Type Conversion13/1  "<meanVelocityZ>"
  Bus Selector2/9 -> Data Type Conversion18/1  "<beamDistance4>"
  Bus Selector2/5 -> Data Type Conversion14/1  "<velocityZ2>"
  Bus Selector2/6 -> Data Type Conversion20/1  "<beamDistance1>"
  Bus Selector2/7 -> Data Type Conversion16/1  "<beamDistance2>"
  Bus Selector2/8 -> Data Type Conversion19/1  "<beamDistance3>"
  Bus Selector2/4 -> Data Type Conversion15/1  "<velocityZ1>"
  Bus Selector2/3 -> Data Type Conversion12/1  "<velocityY>"
  Bus Selector2/2 -> Data Type Conversion17/1  "<velocityX>"
  Bus Selector2/1 -> Data Type Conversion11/1  "<timestampUTC>"
  Byte Pack1/1 -> Vector Concatenate/2
  Data Type Conversion5/1 -> Convert Single Network Byte Order/1
  Convert Single Network Byte Order/1 -> Byte Pack/2
  Data Type Conversion1/1 -> Convert Single Network Byte Order1/1
  Data Type Conversion2/1 -> Convert Single Network Byte Order3/1
  Data Type Conversion3/1 -> Convert Single Network Byte Order2/1
  Data Type Conversion7/1 -> Convert Single Network Byte Order6/1
  Data Type Conversion6/1 -> Convert Single Network Byte Order7/1
  Data Type Conversion4/1 -> Convert Single Network Byte Order5/1
  Data Type Conversion8/1 -> Convert Single Network Byte Order4/1
  Data Type Conversion9/1 -> Convert Single Network Byte Order9/1
  Data Type Conversion10/1 -> Convert Single Network Byte Order8/1
  Convert Single Network Byte Order1/1 -> Byte Pack/3
  Convert Single Network Byte Order2/1 -> Byte Pack/4
  Convert Single Network Byte Order3/1 -> Byte Pack/5
  Convert Single Network Byte Order4/1 -> Byte Pack/6
  Convert Single Network Byte Order5/1 -> Byte Pack/7
  Convert Single Network Byte Order6/1 -> Byte Pack/8
  Convert Single Network Byte Order7/1 -> Byte Pack/9
  Convert Single Network Byte Order8/1 -> Byte Pack/10
  Convert Single Network Byte Order9/1 -> Byte Pack/11
  Convert Single Network Byte Order19/1 -> Byte Pack1/11
  Convert Single Network Byte Order18/1 -> Byte Pack1/10
  Convert Single Network Byte Order17/1 -> Byte Pack1/9
  Convert Single Network Byte Order16/1 -> Byte Pack1/8
  Convert Single Network Byte Order15/1 -> Byte Pack1/7
  Convert Single Network Byte Order14/1 -> Byte Pack1/6
  Convert Single Network Byte Order13/1 -> Byte Pack1/5
  Convert Single Network Byte Order12/1 -> Byte Pack1/4
  Convert Single Network Byte Order11/1 -> Byte Pack1/3
  Data Type Conversion13/1 -> Convert Single Network Byte Order18/1
  Data Type Conversion21/1 -> Convert Single Network Byte Order19/1
  Data Type Conversion20/1 -> Convert Single Network Byte Order14/1
  Data Type Conversion16/1 -> Convert Single Network Byte Order15/1
  Data Type Conversion18/1 -> Convert Single Network Byte Order17/1
  Data Type Conversion19/1 -> Convert Single Network Byte Order16/1
  Data Type Conversion15/1 -> Convert Single Network Byte Order12/1
  Data Type Conversion14/1 -> Convert Single Network Byte Order13/1
  Data Type Conversion12/1 -> Convert Single Network Byte Order11/1
  Convert Single Network Byte Order10/1 -> Byte Pack1/2
  Data Type Conversion17/1 -> Convert Single Network Byte Order10/1
  Convert Double Network Byte Order1/1 -> Byte Pack1/1
  Data Type Conversion11/1 -> Convert Double Network Byte Order1/1

== system MESSIN_Library/State Message/Pack MESSIN State Message/Pack ExternCommand ==
  externCommand : Inport
  Bus Selector : BusSelector  OutputSignals=actuatorCommand
  Bus Selector1 : BusSelector  OutputSignals=allocationCommand
  Pack ActuatorCommand : Subsystem
  Pack AllocationCommand : Subsystem
  Pack Info : Subsystem
  Vector Concatenate : Concatenate  NumInputs=3
  bytes : Outport
  wires:
  Pack ActuatorCommand/1(bytes) -> Vector Concatenate/2
  Pack Info/1(bytes) -> Vector Concatenate/1
  Pack AllocationCommand/1(bytes) -> Vector Concatenate/3
  Vector Concatenate/1 -> bytes/1
  externCommand/1 -> Pack Info/1(externCommand), Bus Selector1/1, Bus Selector/1
  Bus Selector/1 -> Pack ActuatorCommand/1(actuatorCommand)  "<actuatorCommand>"
  Bus Selector1/1 -> Pack AllocationCommand/1(allocationCommand)  "<allocationCommand>"

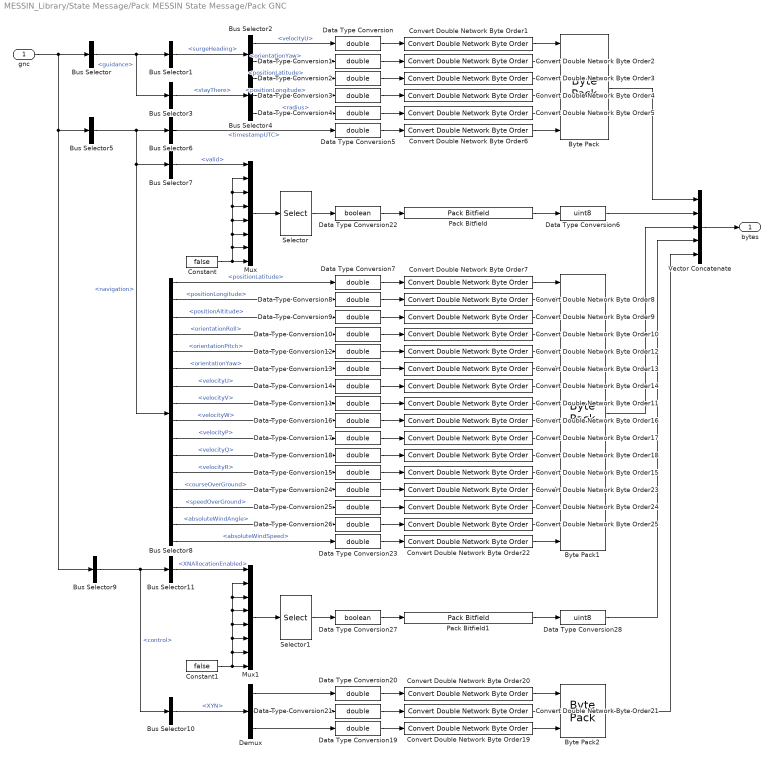
== system MESSIN_Library/State Message/Pack MESSIN State Message/Pack GNC ==
  gnc : Inport
  Bus Selector : BusSelector  OutputSignals=guidance
  Bus Selector1 : BusSelector  OutputSignals=surgeHeading
  Bus Selector10 : BusSelector  OutputSignals=XYN
  Bus Selector11 : BusSelector  OutputSignals=XNAllocationEnabled
  Bus Selector2 : BusSelector  OutputSignals=velocityU,orientationYaw
  Bus Selector3 : BusSelector  OutputSignals=stayThere
  Bus Selector4 : BusSelector  OutputSignals=positionLatitude,positionLongitude,radius
  Bus Selector5 : BusSelector  OutputSignals=navigation
  Bus Selector6 : BusSelector  OutputSignals=timestampUTC
  Bus Selector7 : BusSelector  OutputSignals=info.valid
  Bus Selector8 : BusSelector  OutputSignals=state.positionLatitude,state.positionLongitude,state.positionAltitude,state.orientationRoll,state.orientationPitch,state.orientationYaw,state.velocityU,state.velocityV,state.velocityW,state.velocityP,state.velocityQ,state.velocityR,state.courseOverGround,state.speedOverGround,state.absoluteWindAngle,state.absoluteWindSpeed
  Bus Selector9 : BusSelector  OutputSignals=control
  Byte Pack : etargetslib/Byte Pack  datatypes={'double','double','double','double','double','double'}  byteAlign=1
  Byte Pack1 : etargetslib/Byte Pack  datatypes={'double','double','double','double','double','double','double','double','double','double','double','double','double','double','double','double'}  byteAlign=1
  Byte Pack2 : etargetslib/Byte Pack  datatypes={'double','double','double'}  byteAlign=1
  Constant : Constant  Value=false  OutDataTypeStr=boolean
  Constant1 : Constant  Value=false  OutDataTypeStr=boolean
  Convert Double Network Byte Order{1..25} (25 alike) : $bdroot/Utilities/Convert Double Network Byte Order
  Data Type Conversion{,1..5,7..21,23..26} (25 alike) : DataTypeConversion  OutDataTypeStr=double  SaturateOnIntegerOverflow=off  RndMeth=Floor
  Data Type Conversion22 : DataTypeConversion  OutDataTypeStr=boolean  SaturateOnIntegerOverflow=off  RndMeth=Floor
  Data Type Conversion27 : DataTypeConversion  OutDataTypeStr=boolean  SaturateOnIntegerOverflow=off  RndMeth=Floor
  Data Type Conversion28 : DataTypeConversion  OutDataTypeStr=uint8  SaturateOnIntegerOverflow=off  RndMeth=Floor
  Data Type Conversion6 : DataTypeConversion  OutDataTypeStr=uint8  SaturateOnIntegerOverflow=off  RndMeth=Floor
  Demux : Demux  Outputs=3
  Mux : Mux  Inputs=8
  Mux1 : Mux  Inputs=8
  Pack Bitfield : $bdroot/Utilities/Pack Bitfield
  Pack Bitfield1 : $bdroot/Utilities/Pack Bitfield
  Selector : Selector  InputPortWidth=8  IndexOptions=Index vector (dialog)  Indices=[8 7 6 5 4 3 2 1]  OutputSizes=1
  Selector1 : Selector  InputPortWidth=8  IndexOptions=Index vector (dialog)  Indices=[8 7 6 5 4 3 2 1]  OutputSizes=1
  Vector Concatenate : Concatenate  NumInputs=5
  bytes : Outport
  wires:
  Byte Pack/1 -> Vector Concatenate/1
  Data Type Conversion/1 -> Convert Double Network Byte Order1/1
  gnc/1 -> Bus Selector9/1, Bus Selector5/1, Bus Selector/1
  Bus Selector/1 -> Bus Selector3/1, Bus Selector1/1  "<guidance>"
  Bus Selector1/1 -> Bus Selector2/1  "<surgeHeading>"
  Bus Selector2/1 -> Data Type Conversion/1  "<velocityU>"
  Data Type Conversion1/1 -> Convert Double Network Byte Order2/1
  Bus Selector2/2 -> Data Type Conversion1/1  "<orientationYaw>"
  Bus Selector3/1 -> Bus Selector4/1  "<stayThere>"
  Data Type Conversion2/1 -> Convert Double Network Byte Order3/1
  Data Type Conversion4/1 -> Convert Double Network Byte Order5/1
  Data Type Conversion3/1 -> Convert Double Network Byte Order4/1
  Bus Selector4/1 -> Data Type Conversion2/1  "<positionLatitude>"
  Bus Selector4/2 -> Data Type Conversion3/1  "<positionLongitude>"
  Bus Selector4/3 -> Data Type Conversion4/1  "<radius>"
  Bus Selector5/1 -> Bus Selector8/1, Bus Selector7/1, Bus Selector6/1  "<navigation>"
  Data Type Conversion5/1 -> Convert Double Network Byte Order6/1
  Bus Selector6/1 -> Data Type Conversion5/1  "<timestampUTC>"
  Bus Selector7/1 -> Mux/1  "<valid>"
  Pack Bitfield/1 -> Data Type Conversion6/1
  Mux/1 -> Selector/1
  Constant/1 -> Mux/7, Mux/5, Mux/4, Mux/3, Mux/2, Mux/6, Mux/8
  Convert Double Network Byte Order1/1 -> Byte Pack/1
  Convert Double Network Byte Order2/1 -> Byte Pack/2
  Convert Double Network Byte Order3/1 -> Byte Pack/3
  Convert Double Network Byte Order4/1 -> Byte Pack/4
  Convert Double Network Byte Order5/1 -> Byte Pack/5
  Convert Double Network Byte Order6/1 -> Byte Pack/6
  Data Type Conversion6/1 -> Vector Concatenate/2
  Data Type Conversion7/1 -> Convert Double Network Byte Order7/1
  Bus Selector8/1 -> Data Type Conversion7/1  "<positionLatitude>"
  Data Type Conversion8/1 -> Convert Double Network Byte Order8/1
  Data Type Conversion10/1 -> Convert Double Network Byte Order10/1
  Data Type Conversion9/1 -> Convert Double Network Byte Order9/1
  Data Type Conversion14/1 -> Convert Double Network Byte Order14/1
  Data Type Conversion11/1 -> Convert Double Network Byte Order11/1
  Data Type Conversion13/1 -> Convert Double Network Byte Order13/1
  Data Type Conversion12/1 -> Convert Double Network Byte Order12/1
  Bus Selector8/2 -> Data Type Conversion8/1  "<positionLongitude>"
  Bus Selector8/3 -> Data Type Conversion9/1  "<positionAltitude>"
  Bus Selector8/4 -> Data Type Conversion10/1  "<orientationRoll>"
  Bus Selector8/5 -> Data Type Conversion12/1  "<orientationPitch>"
  Bus Selector8/6 -> Data Type Conversion13/1  "<orientationYaw>"
  Bus Selector8/7 -> Data Type Conversion14/1  "<velocityU>"
  Bus Selector8/8 -> Data Type Conversion11/1  "<velocityV>"
  Bus Selector8/12 -> Data Type Conversion15/1  "<velocityR>"
  Bus Selector8/11 -> Data Type Conversion18/1  "<velocityQ>"
  Bus Selector8/10 -> Data Type Conversion17/1  "<velocityP>"
  Bus Selector8/9 -> Data Type Conversion16/1  "<velocityW>"
  Data Type Conversion16/1 -> Convert Double Network Byte Order16/1
  Data Type Conversion17/1 -> Convert Double Network Byte Order17/1
  Data Type Conversion15/1 -> Convert Double Network Byte Order15/1
  Data Type Conversion18/1 -> Convert Double Network Byte Order18/1
  Convert Double Network Byte Order7/1 -> Byte Pack1/1
  Convert Double Network Byte Order8/1 -> Byte Pack1/2
  Convert Double Network Byte Order9/1 -> Byte Pack1/3
  Convert Double Network Byte Order10/1 -> Byte Pack1/4
  Convert Double Network Byte Order12/1 -> Byte Pack1/5
  Convert Double Network Byte Order13/1 -> Byte Pack1/6
  Convert Double Network Byte Order14/1 -> Byte Pack1/7
  Convert Double Network Byte Order11/1 -> Byte Pack1/8
  Convert Double Network Byte Order16/1 -> Byte Pack1/9
  Byte Pack1/1 -> Vector Concatenate/3
  Vector Concatenate/1 -> bytes/1
  Bus Selector9/1 -> Bus Selector10/1, Bus Selector11/1  "<control>"
  Bus Selector10/1 -> Demux/1  "<XYN>"
  Data Type Conversion21/1 -> Convert Double Network Byte Order21/1
  Data Type Conversion19/1 -> Convert Double Network Byte Order19/1
  Data Type Conversion20/1 -> Convert Double Network Byte Order20/1
  Demux/1 -> Data Type Conversion20/1
  Demux/2 -> Data Type Conversion21/1
  Demux/3 -> Data Type Conversion19/1
  Selector/1 -> Data Type Conversion22/1
  Data Type Conversion22/1 -> Pack Bitfield/1
  Data Type Conversion26/1 -> Convert Double Network Byte Order25/1
  Data Type Conversion23/1 -> Convert Double Network Byte Order22/1
  Data Type Conversion25/1 -> Convert Double Network Byte Order24/1
  Data Type Conversion24/1 -> Convert Double Network Byte Order23/1
  Bus Selector8/13 -> Data Type Conversion24/1  "<courseOverGround>"
  Bus Selector8/14 -> Data Type Conversion25/1  "<speedOverGround>"
  Bus Selector8/15 -> Data Type Conversion26/1  "<absoluteWindAngle>"
  Bus Selector8/16 -> Data Type Conversion23/1  "<absoluteWindSpeed>"
  Convert Double Network Byte Order17/1 -> Byte Pack1/10
  Convert Double Network Byte Order18/1 -> Byte Pack1/11
  Convert Double Network Byte Order15/1 -> Byte Pack1/12
  Convert Double Network Byte Order23/1 -> Byte Pack1/13
  Convert Double Network Byte Order24/1 -> Byte Pack1/14
  Convert Double Network Byte Order25/1 -> Byte Pack1/15
  Convert Double Network Byte Order22/1 -> Byte Pack1/16
  Convert Double Network Byte Order20/1 -> Byte Pack2/1
  Convert Double Network Byte Order21/1 -> Byte Pack2/2
  Convert Double Network Byte Order19/1 -> Byte Pack2/3
  Data Type Conversion27/1 -> Pack Bitfield1/1
  Selector1/1 -> Data Type Conversion27/1
  Constant1/1 -> Mux1/8, Mux1/6, Mux1/2, Mux1/3, Mux1/4, Mux1/5, Mux1/7
  Mux1/1 -> Selector1/1
  Pack Bitfield1/1 -> Data Type Conversion28/1
  Bus Selector11/1 -> Mux1/1  "<XNAllocationEnabled>"
  Data Type Conversion28/1 -> Vector Concatenate/4
  Byte Pack2/1 -> Vector Concatenate/5

== system MESSIN_Library/State Message/Pack MESSIN State Message/Pack GNSS ==
  gnss : Inport
  Bus Selector1 : BusSelector  OutputSignals=courseAndSpeedOverGround
  Bus Selector2 : BusSelector  OutputSignals=timestampUTC,courseOverGround,speedOverGround
  Bus Selector3 : BusSelector  OutputSignals=gnss
  Bus Selector4 : BusSelector  OutputSignals=timestampUTC,latitude,longitude,altitude,hdop,numSat,gpsQuality
  Byte Pack1 : S-Function  FunctionName=any2byte  Parameters=datatypesout,byteAlign  SFunctionDeploymentMode=off  EnableBusSupport=off  mask(Byte pack){datatypes={'double','single','single'}, byteAlign=1}
      mask prompts: datatypes "Input port data types (cell array):"; byteAlign "Byte alignment:"
      mask help: Pack input data into a single output vector of type uint8. Insert before a UDP Send block to produce a uint8 byte vector from multiple vectors of varying data type.
      mask init:
      | datatypesout = bytepack_callback(datatypes);
      settings: LibrarySourceBlock=embeddedtargetslib/Host Communication/Byte Pack
      mask Help: eval('linkfoundation.util.openBlockHelp(''etargetslibbytepack'')');
      mask TypeOptions byteAlign: 1 | 2 | 4 | 8
      mask Display:
      | color('blue');
      | text(0.95, 0.90, '', ...
      |                 'horizontalalignment', 'right');
      | color('black');
      | text(0.50, 0.12, 'Byte Pack', ...
      |                 'horizontalAlignment','center');
  Byte Pack2 : S-Function  FunctionName=any2byte  Parameters=datatypesout,byteAlign  SFunctionDeploymentMode=off  EnableBusSupport=off  mask(Byte pack){datatypes={'double','double','double','single','single','uint8','uint8'}, byteAlign=1}
      mask prompts: datatypes "Input port data types (cell array):"; byteAlign "Byte alignment:"
      mask help: Pack input data into a single output vector of type uint8. Insert before a UDP Send block to produce a uint8 byte vector from multiple vectors of varying data type.
      mask init:
      | datatypesout = bytepack_callback(datatypes);
      settings: LibrarySourceBlock=embeddedtargetslib/Host Communication/Byte Pack
      mask Help: eval('linkfoundation.util.openBlockHelp(''etargetslibbytepack'')');
      mask TypeOptions byteAlign: 1 | 2 | 4 | 8
      mask Display:
      | color('blue');
      | text(0.95, 0.90, '', ...
      |                 'horizontalalignment', 'right');
      | color('black');
      | text(0.50, 0.12, 'Byte Pack', ...
      |                 'horizontalAlignment','center');
  Convert Double Network Byte Order{,2..4} (4 alike) : $bdroot/Utilities/Convert Double Network Byte Order
  Convert Single Network Byte Order{,1..3} (4 alike) : $bdroot/Utilities/Convert Single Network Byte Order
  Data Type Conversion{1..2,5..6} (4 alike) : DataTypeConversion  OutDataTypeStr=double  SaturateOnIntegerOverflow=off  RndMeth=Floor
  Data Type Conversion{3..4,7,11} (4 alike) : DataTypeConversion  OutDataTypeStr=single  SaturateOnIntegerOverflow=off  RndMeth=Floor
  Data Type Conversion12 : DataTypeConversion  OutDataTypeStr=uint8  SaturateOnIntegerOverflow=off  RndMeth=Floor
  Data Type Conversion8 : DataTypeConversion  OutDataTypeStr=uint8  SaturateOnIntegerOverflow=off  RndMeth=Floor
  Vector Concatenate : Concatenate
  bytes : Outport
  wires:
  Data Type Conversion12/1 -> Byte Pack2/7
  Convert Single Network Byte Order/1 -> Byte Pack2/4
  Convert Double Network Byte Order4/1 -> Byte Pack2/3
  Convert Double Network Byte Order3/1 -> Byte Pack2/2
  Convert Double Network Byte Order2/1 -> Byte Pack2/1
  Data Type Conversion7/1 -> Convert Single Network Byte Order/1
  Data Type Conversion6/1 -> Convert Double Network Byte Order4/1
  Data Type Conversion5/1 -> Convert Double Network Byte Order3/1
  Bus Selector4/7 -> Data Type Conversion12/1  "<gpsQuality>"
  Bus Selector4/5 -> Data Type Conversion11/1  "<hdop>"
  Bus Selector4/6 -> Data Type Conversion8/1  "<numSat>"
  Bus Selector4/4 -> Data Type Conversion7/1  "<altitude>"
  Bus Selector4/3 -> Data Type Conversion6/1  "<longitude>"
  Bus Selector4/2 -> Data Type Conversion5/1  "<latitude>"
  Bus Selector4/1 -> Data Type Conversion2/1  "<timestampUTC>"
  Data Type Conversion2/1 -> Convert Double Network Byte Order2/1
  Bus Selector3/1 -> Bus Selector4/1  "<gnss>"
  Vector Concatenate/1 -> bytes/1
  gnss/1 -> Bus Selector1/1, Bus Selector3/1
  Bus Selector2/3 -> Data Type Conversion3/1  "<speedOverGround>"
  Bus Selector2/2 -> Data Type Conversion4/1  "<courseOverGround>"
  Bus Selector2/1 -> Data Type Conversion1/1  "<timestampUTC>"
  Convert Double Network Byte Order/1 -> Byte Pack1/1
  Data Type Conversion1/1 -> Convert Double Network Byte Order/1
  Bus Selector1/1 -> Bus Selector2/1  "<courseAndSpeedOverGround>"
  Data Type Conversion11/1 -> Convert Single Network Byte Order1/1
  Convert Single Network Byte Order1/1 -> Byte Pack2/5
  Data Type Conversion8/1 -> Byte Pack2/6
  Byte Pack2/1 -> Vector Concatenate/1
  Byte Pack1/1 -> Vector Concatenate/2
  Data Type Conversion3/1 -> Convert Single Network Byte Order3/1
  Data Type Conversion4/1 -> Convert Single Network Byte Order2/1
  Convert Single Network Byte Order2/1 -> Byte Pack1/2
  Convert Single Network Byte Order3/1 -> Byte Pack1/3

== system MESSIN_Library/State Message/Pack MESSIN State Message/Pack Header ==
  note: M essin S tate
  ID : Constant  Value=uint8('MS')  OutDataTypeStr=uint8
  bytes : Outport
  wires:
  ID/1 -> bytes/1
